simulink model "cart_pendulum"  (R2023b)
settings: Solver=VariableStepAuto  StartTime=0.0  StopTime=2  RelTol=1e-3
values from neighbouring files (symbols this model uses):
  g = 9.8    [param_for_cart.m]
  l = 0.5    [param_for_cart.m]
  m = 0.5    [param_for_cart.m]
  M = 1    [param_for_cart.m]
libraries: simulink x3
settings Model: Creator=zhy  LastModifiedBy=zhy

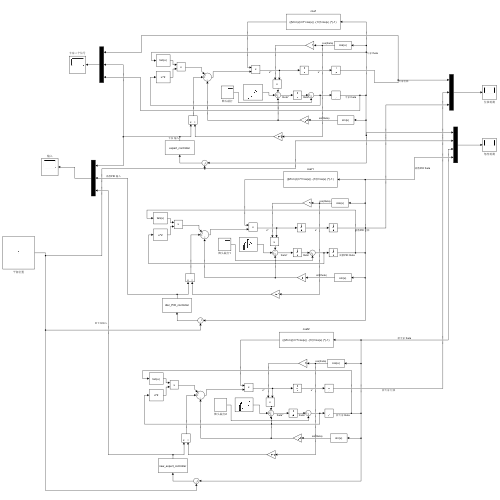
[thumbnail: Simulink's stored preview of the top-level diagram]
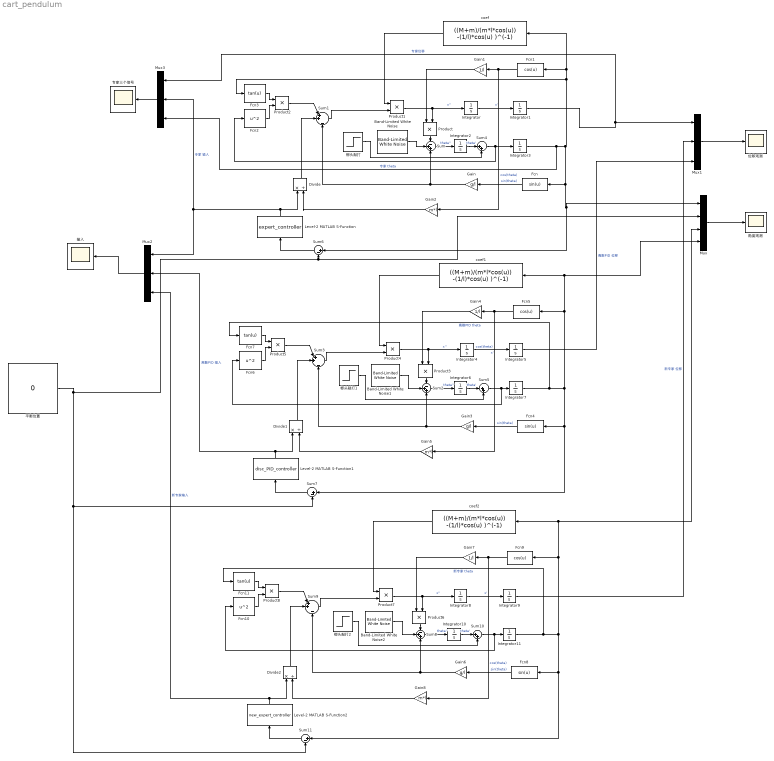
== system cart_pendulum ==
  Band-Limited White Noise : simulink/Sources/Band-Limited White Noise  Cov=[0.1]  Ts=0.00001  seed=[23341]
  Band-Limited White Noise1 : simulink/Sources/Band-Limited White Noise  Cov=[0.1]  Ts=0.00001  seed=[23341]
  Band-Limited White Noise2 : simulink/Sources/Band-Limited White Noise  Cov=[0.1]  Ts=0.00001  seed=[23341]
  Divide : Product  Inputs=*/
  Divide1 : Product  Inputs=*/
  Divide2 : Product  Inputs=*/
  Fcn : Fcn  Expr=sin(u)
  Fcn1 : Fcn  Expr=cos(u)
  Fcn10 : Fcn  Expr=u^2
  Fcn11 : Fcn  Expr=tan(u)
  Fcn2 : Fcn  Expr=u^2
  Fcn3 : Fcn  Expr=tan(u)
  Fcn4 : Fcn  Expr=sin(u)
  Fcn5 : Fcn  Expr=cos(u)
  Fcn6 : Fcn  Expr=u^2
  Fcn7 : Fcn  Expr=tan(u)
  Fcn8 : Fcn  Expr=sin(u)
  Fcn9 : Fcn  Expr=cos(u)
  Gain : Gain  Gain=g/l
  Gain1 : Gain  Gain=1/l
  Gain2 : Gain  Gain=m*l
  Gain3 : Gain  Gain=g/l
  Gain4 : Gain  Gain=1/l
  Gain5 : Gain  Gain=m*l
  Gain6 : Gain  Gain=g/l
  Gain7 : Gain  Gain=1/l
  Gain8 : Gain  Gain=m*l
  Integrator{,1..2,4..6,8..10} (9 alike) : Integrator
  Integrator11 : Integrator  InitialCondition=pi/4
  Integrator3 : Integrator  InitialCondition=0.25*pi
  Integrator7 : Integrator  InitialCondition=pi/4
  Level-2 MATLAB S-Function : M-S-Function  FunctionName=expert_controller  Parameters=0,0,0
  Level-2 MATLAB S-Function1 : M-S-Function  FunctionName=disc_PID_controller  Parameters=0,0,0
  Level-2 MATLAB S-Function2 : M-S-Function  FunctionName=new_expert_controller  Parameters=0,0,0
  Mux : Mux
  Mux1 : Mux  Inputs=3
  Mux2 : Mux  Inputs=3
  Mux3 : Mux  Inputs=3
  Product{,1..8} (9 alike) : Product
  Sum : Sum  Inputs=-++
  Sum1 : Sum  Inputs=|++|-
  Sum10 : Sum  Inputs=|++
  Sum11 : Sum  Inputs=|+-
  Sum2 : Sum  Inputs=-++
  Sum3 : Sum  Inputs=|++|-
  Sum4 : Sum  Inputs=|++
  Sum5 : Sum  Inputs=|++
  Sum6 : Sum  Inputs=|+-
  Sum7 : Sum  Inputs=|+-
  Sum8 : Sum  Inputs=-++
  Sum9 : Sum  Inputs=|++|-
  coef : Fcn  Expr=((M+m)/(m*l*cos(u)) -(1/l)*cos(u) )^(-1)
  coef1 : Fcn  Expr=((M+m)/(m*l*cos(u)) -(1/l)*cos(u) )^(-1)
  coef2 : Fcn  Expr=((M+m)/(m*l*cos(u)) -(1/l)*cos(u) )^(-1)
  专家三个信号 : Scope
  位移观测 : Scope
  平衡位置 : Constant  Value=0
  榔头敲打 : Step  Time=0.8  After=0  SampleTime=0
  榔头敲打1 : Step  Time=0.8  After=0  SampleTime=0
  榔头敲打2 : Step  Time=0  After=pi  SampleTime=0
  角度观测 : Scope
  输入 : Scope
  wires:
  Integrator/1 -> Integrator1/1  "x'"
  Fcn/1 -> Gain/1  "sin(theta)"
  Sum/1 -> Integrator2/1  "theta''"
  Gain/1 -> Sum/3, Sum1/3
  Product/1 -> Sum/1
  Product1/1 -> Integrator/1, Product/2  "x''"
  Fcn1/1 -> Gain1/1, Gain2/1  "cos(theta)"
  Gain1/1 -> Product/1
  coef/1 -> Product1/1
  Fcn3/1 -> Product2/1
  Fcn2/1 -> Product2/2
  Product2/1 -> Sum1/1
  Level-2 MATLAB S-Function/1 -> Divide/1, Mux3/2, Mux2/1  "专家 输入"
  Divide/1 -> Sum1/2
  Gain2/1 -> Divide/2
  Sum1/1 -> Product1/2
  Integrator5/1 -> Mux1/3  "离散PID 位移"
  Level-2 MATLAB S-Function1/1 -> Divide1/1, Mux2/2  "离散PID 输入"
  coef1/1 -> Product4/1
  Product4/1 -> Integrator4/1, Product3/2  "x''"
  Fcn6/1 -> Product5/2
  Fcn4/1 -> Gain3/1  "sin(theta)"
  Fcn5/1 -> Gain4/1, Gain5/1  "cos(theta)"
  Divide1/1 -> Sum3/2
  Sum3/1 -> Product4/2
  Product5/1 -> Sum3/1
  Fcn7/1 -> Product5/1
  Gain5/1 -> Divide1/2
  Gain3/1 -> Sum2/3, Sum3/3
  Product3/1 -> Sum2/1
  Integrator7/1 -> Fcn7/1, Mux/4, coef1/1, Fcn5/1, Sum7/1, Fcn4/1  "离散PID theta"
  Gain4/1 -> Product3/1
  Integrator4/1 -> Integrator5/1  "x'"
  Sum2/1 -> Integrator6/1  "theta''"
  Mux1/1 -> 位移观测/1
  Mux/1 -> 角度观测/1
  Integrator1/1 -> Mux3/1, Mux1/1  "专家位移"
  Mux2/1 -> 输入/1
  Mux3/1 -> 专家三个信号/1
  Integrator3/1 -> Mux3/3, Sum6/1, Mux/1, Fcn/1, Fcn3/1, coef/1, Fcn1/1  "专家 theta"
  Band-Limited White Noise1/1 -> Sum2/2
  Band-Limited White Noise/1 -> Sum/2
  Integrator2/1 -> Sum4/1  "theta'"
  Sum4/1 -> Fcn2/1, Integrator3/1
  Integrator6/1 -> Sum5/1  "theta'"
  Sum5/1 -> Fcn6/1, Integrator7/1
  榔头敲打/1 -> Sum4/2
  榔头敲打1/1 -> Sum5/2
  Sum6/1 -> Level-2 MATLAB S-Function/1
  平衡位置/1 -> Sum6/2, Mux/2, Sum11/2, Sum7/2
  Sum7/1 -> Level-2 MATLAB S-Function1/1
  Integrator10/1 -> Sum10/1  "theta'"
  榔头敲打2/1 -> Sum10/2
  Integrator11/1 -> Fcn11/1, Mux/3, coef2/1, Fcn9/1, Sum11/1, Fcn8/1  "新专家 theta"
  Sum11/1 -> Level-2 MATLAB S-Function2/1
  Gain8/1 -> Divide2/2
  Product8/1 -> Sum9/1
  Product6/1 -> Sum8/1
  Sum8/1 -> Integrator10/1  "theta''"
  Gain6/1 -> Sum8/3, Sum9/3
  Integrator8/1 -> Integrator9/1  "x'"
  Sum10/1 -> Fcn10/1, Integrator11/1
  Fcn11/1 -> Product8/1
  Sum9/1 -> Product7/2
  Fcn10/1 -> Product8/2
  Fcn8/1 -> Gain6/1  "sin(theta)"
  Fcn9/1 -> Gain7/1, Gain8/1  "cos(theta)"
  Level-2 MATLAB S-Function2/1 -> Mux2/3, Divide2/1  "新专家输入"
  Integrator9/1 -> Mux1/2  "新专家 位移"
  Gain7/1 -> Product6/1
  Divide2/1 -> Sum9/2
  Product7/1 -> Integrator8/1, Product6/2  "x''"
  coef2/1 -> Product7/1
  Band-Limited White Noise2/1 -> Sum8/2
